simulink model "BD_PAR_AUTO_base_model"  (Simulink 10.3)
settings: Solver=ode1  StartTime=0.0  StopTime=max(cyc_mph(:,1))  FixedStep=1  MaxStep=1  RelTol=1e-3  AbsTol=1e-3
undefined symbols (not defined in the file): acc_dcdc_eff, acc_elec_eff, acc_elec_pwr, acc_mech_eff, acc_mech_pwr, acc_mech_trq, air_cp, amb_tmp, cs_charge_deplete_bool, cs_charge_trq, cs_electric_decel_spd, cs_electric_launch_spd_hi, cs_electric_launch_spd_lo, cs_hi_soc, cs_lo_soc, cs_min_trq_frac, cs_off_trq_frac, cyc_avg_time, cyc_cargo_mass, cyc_elevation_init, cyc_filter_bool, cyc_grade, cyc_mph, enable_sim_stop_distance, enable_sim_stop_max_spd, enable_sim_stop_speed, enable_sim_stop_time, enable_stop, enable_stop_fc, ess_cap_scale, ess_coulombic_eff, ess_init_soc, ess_max_ah_cap, ess_max_volts, ess_min_volts, ess_mod_airflow, ess_mod_cp, ess_mod_init_tmp, ess_module_mass, ess_module_num, ess_on, ess_r_chg, ess_r_dis, ess_res_scale_coef, ess_res_scale_fun, ess_set_tmp, ess_soc, ess_th_calc, ess_th_res_off, ess_th_res_on, ess_tmp, ess_voc, ex_calc, ex_cat_co_frac, ex_cat_ext_cp, ex_cat_ext_emisv, ex_cat_ext_init_tmp, ex_cat_ext_mass, ex_cat_ext_sarea, ex_cat_hc_frac ... (+168)
(part 8 of 15)

== system BD_PAR_AUTO_base_model/<vc> par auto/gearbox control for use w/ AT/shifting1/time since last shift/just shifted ==
  in_1 : Inport
  Memory : Memory  InitialCondition=1
  Relational Operator : RelationalOperator  Operator=~=  RndMeth=Nearest  InputSameDT=on
  out_1 : Outport  InitialOutput=0
  wires:
  in_1/1 -> Memory/1, Relational Operator/2
  Memory/1 -> Relational Operator/1
  Relational Operator/1 -> out_1/1

== system BD_PAR_AUTO_base_model/<vc> par auto/gearbox control for use w/ AT/shifting1/time since last shift/timer ==
  trigger : Inport
  Constant : Constant
  Constant1 : Constant  Value=0
  Constant2 : Constant  Value=0
  Switch : Switch  Threshold=eps
  no-lag Reset Integrator : Subsystem  mask(No-lag Reset Integrator){initval=15}
      mask prompts: initval "Initial Value"
      mask help: No-lag Reset Integrator
      mask Help: Integrates first input using Euler technique.\nAt the time step that input 2 <> zero,\noutput is reset to input 3.
      mask Display: disp('1/s\nw/ reset\nno lag')
  time : Outport  InitialOutput=0
  wires:
  no-lag Reset Integrator/1(out_1) -> Switch/3
  Constant1/1 -> no-lag Reset Integrator/3(in_3)
  Constant/1 -> no-lag Reset Integrator/1(in_1)
  Constant2/1 -> Switch/1
  trigger/1 -> no-lag Reset Integrator/2(in_2), Switch/2
  Switch/1 -> time/1

== system BD_PAR_AUTO_base_model/electric acc loads <acc>/Electrical Accessory Loads v2 <acc>/backward model/electrical accessories (W)/Electrical Accessories: Time Variable ==
  note: (W)
  Constant : Constant  Value=acc_elec_pwr
  Constant1 : Constant  Value=load_on
  Elec Aux Loads 14V Pwr : Subsystem
  Elec Aux Loads HiV Pwr : Subsystem
  Product : Product  InputSameDT=on  RndMeth=Zero  SaturateOnIntegerOverflow=on  OutDataTypeStr=Inherit: Same as first input
  Sum : Sum  Inputs=+++  InputSameDT=on  SaturateOnIntegerOverflow=on  OutDataTypeStr=Inherit: Same as first input
  dcdc converter : Gain  Gain=1/acc_dcdc_eff  SaturateOnIntegerOverflow=on  OutDataTypeStr=Inherit: Same as input  ParamDataTypeStr=Inherit: Same as input
  divide by eff : Gain  Gain=1/acc_elec_eff  SaturateOnIntegerOverflow=on  OutDataTypeStr=Inherit: Same as input  ParamDataTypeStr=Inherit: Same as input
  P_elec_acc : Outport  InitialOutput=0
  wires:
  Elec Aux Loads HiV Pwr/1(Out1) -> Sum/3
  dcdc converter/1 -> Sum/2
  Constant/1 -> Sum/1
  Constant1/1 -> Product/2
  Product/1 -> P_elec_acc/1
  divide by eff/1 -> Product/1
  Sum/1 -> divide by eff/1
  Elec Aux Loads 14V Pwr/1(Out1) -> dcdc converter/1

== system BD_PAR_AUTO_base_model/energy storage <ess>/ess config/energy storage <ess>/ess tmp/Block NOTES ==
  note: This block models the thermal behavior of a battery module with active air cooling.
      | The module is modeled as a single lumped thermal mass.
      | The fan is on whenever the battery temp is > the set temp.

== system BD_PAR_AUTO_base_model/energy storage <ess>/ess config/energy storage <ess>/ess tmp/Tair,ave ==
  Qess_case : Inport
  Qess_case1 : Inport  Port=2
  Enable : EnablePort  StatesWhenEnabling=reset
  Block NOTES : Subsystem
      mask Display: disp('Block\nNOTES')
  Tamb-(Q/mcp)/1 : Fcn  Expr=amb_tmp - (u(1)/(ess_mod_airflow*air_cp))/2
  Tamb-(Q/mcp)/2 : Fcn  Expr=amb_tmp - (u(1)/(ess_mod_airflow*air_cp))/2
  do ex calcs?1 : Constant  Value=ess_th_res_on
  Tair_ave : Outport  OutputWhenDisabled=reset  InitialOutput=amb_tmp
  Th Res : Outport  Port=2  OutputWhenDisabled=reset  InitialOutput=ess_th_res_off
  Tair : Outport  Port=3  InitialOutput=amb_tmp
  wires:
  Tamb-(Q/mcp)/1/1 -> Tair/1
  Qess_case1/1 -> Tamb-(Q/mcp)/1/1
  Tamb-(Q/mcp)/2/1 -> Tair_ave/1
  Qess_case/1 -> Tamb-(Q/mcp)/2/1
  do ex calcs?1/1 -> Th Res/1

== system BD_PAR_AUTO_base_model/energy storage <ess>/ess config/energy storage <ess>/limit power/Limits ==
  SOC  high limited : Inport
  not SOC  low limited : Inport  Port=2
  power req : Inport  Port=3
  power bat limited : Inport  Port=4
  V used : Inport  Port=5
  V mc_min_volts : Inport  Port=6
  V battery (.5Voc) : Inport  Port=7
  V ess_min_volts : Inport  Port=8
  Logical Operator1 : Logic  Operator=NOT  Inputs=1
  Relational Operator{1,3..5} (4 alike) : RelationalOperator  Operator===  RndMeth=Nearest  InputSameDT=on
  limited by battery : Logic
  limited by battery min V : Logic
  limited by motor controller : Logic
  tag scope: ess_minV_limited=global, ess_pwr_limited=global, ess_soc_hi_limited=global, ess_soc_low_limited=global, mc_voltage_limited=global
  wires:
  power bat limited/1 -> Relational Operator1/2
  V mc_min_volts/1 -> Relational Operator3/2
  V used/1 -> Relational Operator3/1, Relational Operator4/1, Relational Operator5/1
  V battery (.5Voc)/1 -> Relational Operator4/2
  V ess_min_volts/1 -> Relational Operator5/2
  limited by motor controller/1 -> [mc_voltage_limited]
  limited by battery/1 -> [ess_pwr_limited]
  limited by battery min V/1 -> [ess_minV_limited]
  Relational Operator3/1 -> limited by motor controller/2
  Relational Operator1/1 -> limited by motor controller/1, limited by battery/1, limited by battery min V/1
  Relational Operator4/1 -> limited by battery/2
  Relational Operator5/1 -> limited by battery min V/2
  power req/1 -> Relational Operator1/1
  Logical Operator1/1 -> [ess_soc_low_limited]
  not SOC  low limited/1 -> Logical Operator1/1
  SOC  high limited/1 -> [ess_soc_hi_limited]

== system BD_PAR_AUTO_base_model/energy storage <ess>/ess config/energy storage <ess>/max pack pwr (W)1/Rchg (ohms)1 ==
  x0 : Inport
  y0 : Inport  Port=2
  Mux : Mux  Inputs=2
  S-function : S-Function  FunctionName=sftable2  Parameters=xindex, yindex, table  SFunctionDeploymentMode=off  EnableBusSupport=off
  table out : Outport  InitialOutput=0
  wires:
  Mux/1 -> S-function/1
  x0/1 -> Mux/1
  S-function/1 -> table out/1
  y0/1 -> Mux/2

== system BD_PAR_AUTO_base_model/energy storage <ess>/ess config/energy storage <ess>/max pack pwr (W)1/Rdis (ohms) ==
  x0 : Inport
  y0 : Inport  Port=2
  Mux : Mux  Inputs=2
  S-function : S-Function  FunctionName=sftable2  Parameters=xindex, yindex, table  SFunctionDeploymentMode=off  EnableBusSupport=off
  table out : Outport  InitialOutput=0
  wires:
  Mux/1 -> S-function/1
  x0/1 -> Mux/1
  S-function/1 -> table out/1
  y0/1 -> Mux/2

== system BD_PAR_AUTO_base_model/energy storage <ess>/ess config/energy storage <ess>/max pack pwr (W)1/VOC (V) ==
  x0 : Inport
  y0 : Inport  Port=2
  Mux : Mux  Inputs=2
  S-function : S-Function  FunctionName=sftable2  Parameters=xindex, yindex, table  SFunctionDeploymentMode=off  EnableBusSupport=off
  table out : Outport  InitialOutput=0
  wires:
  Mux/1 -> S-function/1
  x0/1 -> Mux/1
  S-function/1 -> table out/1
  y0/1 -> Mux/2

== system BD_PAR_AUTO_base_model/energy storage <ess>/ess config/energy storage <ess>/pack Voc, Rint/Rchg (ohms) ==
  x0 : Inport
  y0 : Inport  Port=2
  Mux : Mux  Inputs=2
  S-function : S-Function  FunctionName=sftable2  Parameters=xindex, yindex, table  SFunctionDeploymentMode=off  EnableBusSupport=off
  table out : Outport  InitialOutput=0
  wires:
  y0/1 -> Mux/2
  S-function/1 -> table out/1
  x0/1 -> Mux/1
  Mux/1 -> S-function/1

== system BD_PAR_AUTO_base_model/energy storage <ess>/ess config/energy storage <ess>/pack Voc, Rint/Rdis (ohms) ==
  x0 : Inport
  y0 : Inport  Port=2
  Mux : Mux  Inputs=2
  S-function : S-Function  FunctionName=sftable2  Parameters=xindex, yindex, table  SFunctionDeploymentMode=off  EnableBusSupport=off
  table out : Outport  InitialOutput=0
  wires:
  y0/1 -> Mux/2
  S-function/1 -> table out/1
  x0/1 -> Mux/1
  Mux/1 -> S-function/1

== system BD_PAR_AUTO_base_model/energy storage <ess>/ess config/energy storage <ess>/pack Voc, Rint/VOC (V) ==
  x0 : Inport
  y0 : Inport  Port=2
  Mux : Mux  Inputs=2
  S-function : S-Function  FunctionName=sftable2  Parameters=xindex, yindex, table  SFunctionDeploymentMode=off  EnableBusSupport=off
  table out : Outport  InitialOutput=0
  wires:
  y0/1 -> Mux/2
  S-function/1 -> table out/1
  x0/1 -> Mux/1
  Mux/1 -> S-function/1

== system BD_PAR_AUTO_base_model/fuel converter  <fc>/engine torque/effect of inertia (Nm)/engine inertia as a function of total vehicle inertia (generous approximation)/veh mass calc ==
  Constant : Constant  Value=veh_mass
  Sum : Sum  Inputs=|++  InputSameDT=on  SaturateOnIntegerOverflow=on  OutDataTypeStr=Inherit: Same as first input
  Out1 : Outport
  wires:
  Sum/1 -> Out1/1
  Constant/1 -> Sum/2
  [veh_cargo_mass] -> Sum/1

== system BD_PAR_AUTO_base_model/fuel converter  <fc>/fuel use and EO emis Configurable Subsystem/fuel use and EO emis/HOT engine maps /Block NOTES ==
  note: This block determines the fully hot fuel use, engine-out emissions output rates, exhaust gas mass flow rate,
      | and engine-out exhaust gas temperature as a function of engine output torque and speed.
      | The engine maps (except for exhaust gas temperature) can be scaled using variables fc_spd_scale and
      |  fc_trq_scale; it is recommended that scaling values outside the range of 0.85 to 1.15 be used CAREFULLY.

== system BD_PAR_AUTO_base_model/fuel converter  <fc>/fuel use and EO emis Configurable Subsystem/fuel use and EO emis/HOT engine maps /CO (g/s) ==
  x0 : Inport
  y0 : Inport  Port=2
  Mux : Mux  Inputs=2
  S-function : S-Function  FunctionName=sftable2  Parameters=xindex, yindex, table  SFunctionDeploymentMode=off  EnableBusSupport=off
  table out : Outport  InitialOutput=0
  wires:
  Mux/1 -> S-function/1
  x0/1 -> Mux/1
  S-function/1 -> table out/1
  y0/1 -> Mux/2

== system BD_PAR_AUTO_base_model/fuel converter  <fc>/fuel use and EO emis Configurable Subsystem/fuel use and EO emis/HOT engine maps /HC (g/s) ==
  x0 : Inport
  y0 : Inport  Port=2
  Mux : Mux  Inputs=2
  S-function : S-Function  FunctionName=sftable2  Parameters=xindex, yindex, table  SFunctionDeploymentMode=off  EnableBusSupport=off
  table out : Outport  InitialOutput=0
  wires:
  Mux/1 -> S-function/1
  x0/1 -> Mux/1
  S-function/1 -> table out/1
  y0/1 -> Mux/2

== system BD_PAR_AUTO_base_model/fuel converter  <fc>/fuel use and EO emis Configurable Subsystem/fuel use and EO emis/HOT engine maps /MF,ex (g/s) ==
  x0 : Inport
  y0 : Inport  Port=2
  Mux : Mux  Inputs=2
  S-function : S-Function  FunctionName=sftable2  Parameters=xindex, yindex, table  SFunctionDeploymentMode=off  EnableBusSupport=off
  table out : Outport  InitialOutput=0
  wires:
  Mux/1 -> S-function/1
  x0/1 -> Mux/1
  S-function/1 -> table out/1
  y0/1 -> Mux/2

== system BD_PAR_AUTO_base_model/fuel converter  <fc>/fuel use and EO emis Configurable Subsystem/fuel use and EO emis/HOT engine maps /NOx (g/s) ==
  x0 : Inport
  y0 : Inport  Port=2
  Mux : Mux  Inputs=2
  S-function : S-Function  FunctionName=sftable2  Parameters=xindex, yindex, table  SFunctionDeploymentMode=off  EnableBusSupport=off
  table out : Outport  InitialOutput=0
  wires:
  Mux/1 -> S-function/1
  x0/1 -> Mux/1
  S-function/1 -> table out/1
  y0/1 -> Mux/2

== system BD_PAR_AUTO_base_model/fuel converter  <fc>/fuel use and EO emis Configurable Subsystem/fuel use and EO emis/HOT engine maps /O2 (g/s) ==
  x0 : Inport
  y0 : Inport  Port=2
  Mux : Mux  Inputs=2
  S-function : S-Function  FunctionName=sftable2  Parameters=xindex, yindex, table  SFunctionDeploymentMode=off  EnableBusSupport=off
  table out : Outport  InitialOutput=0
  wires:
  y0/1 -> Mux/2
  S-function/1 -> table out/1
  x0/1 -> Mux/1
  Mux/1 -> S-function/1

== system BD_PAR_AUTO_base_model/fuel converter  <fc>/fuel use and EO emis Configurable Subsystem/fuel use and EO emis/HOT engine maps /PM (g/s) ==
  x0 : Inport
  y0 : Inport  Port=2
  Mux : Mux  Inputs=2
  S-function : S-Function  FunctionName=sftable2  Parameters=xindex, yindex, table  SFunctionDeploymentMode=off  EnableBusSupport=off
  table out : Outport  InitialOutput=0
  wires:
  Mux/1 -> S-function/1
  x0/1 -> Mux/1
  S-function/1 -> table out/1
  y0/1 -> Mux/2

== system BD_PAR_AUTO_base_model/fuel converter  <fc>/fuel use and EO emis Configurable Subsystem/fuel use and EO emis/HOT engine maps /Tex,eo (C) ==
  x0 : Inport
  y0 : Inport  Port=2
  Mux : Mux  Inputs=2
  S-function : S-Function  FunctionName=sftable2  Parameters=xindex, yindex, table  SFunctionDeploymentMode=off  EnableBusSupport=off
  table out : Outport  InitialOutput=0
  wires:
  Mux/1 -> S-function/1
  x0/1 -> Mux/1
  S-function/1 -> table out/1
  y0/1 -> Mux/2

== system BD_PAR_AUTO_base_model/fuel converter  <fc>/fuel use and EO emis Configurable Subsystem/fuel use and EO emis/HOT engine maps /fuel (g/s) ==
  x0 : Inport
  y0 : Inport  Port=2
  Mux : Mux  Inputs=2
  S-function : S-Function  FunctionName=sftable2  Parameters=xindex, yindex, table  SFunctionDeploymentMode=off  EnableBusSupport=off
  table out : Outport  InitialOutput=0
  wires:
  Mux/1 -> S-function/1
  x0/1 -> Mux/1
  S-function/1 -> table out/1
  y0/1 -> Mux/2

== system BD_PAR_AUTO_base_model/fuel converter  <fc>/fuel use and EO emis Configurable Subsystem/fuel use and EO emis/fc temp/Block NOTES ==
  note: This block models the thermal behavior internal combustion engine (ICE).
      | Emphasis is on the coolant since this temperature is used to correct engine
      | fuel use.

== system BD_PAR_AUTO_base_model/fuel converter  <fc>/fuel use and EO emis Configurable Subsystem/fuel use and EO emis/fc temp/fc coolant ==
  Tcl : Inport
  "Qfc_i " : Inport  Port=2
  Enable : EnablePort  StatesWhenEnabling=reset
  Constant : Constant  Value=fc_tstat
  Product1 : Product  InputSameDT=on  RndMeth=Zero  SaturateOnIntegerOverflow=on  OutDataTypeStr=Inherit: Same as first input
  Qhtr : Fcn  Expr=fc_cl2h_eff*fc_h_air_flow*air_cp*(u - amb_tmp)
  Qi : Sum  Inputs=-+  InputSameDT=on  SaturateOnIntegerOverflow=on  OutDataTypeStr=Inherit: Same as first input
  Relational Operator : RelationalOperator  Operator=<=  RndMeth=Nearest  InputSameDT=on
  Qfc_rad : Outport  OutputWhenDisabled=reset  InitialOutput=0
  Qfc_htr : Outport  Port=2  OutputWhenDisabled=reset  InitialOutput=0
  wires:
  Tcl/1 -> Qhtr/1, Relational Operator/2
  Relational Operator/1 -> Product1/1
  Constant/1 -> Relational Operator/1
  Product1/1 -> Qfc_rad/1
  "Qfc_i "/1 -> Qi/2
  Qhtr/1 -> Qi/1, Qfc_htr/1
  Qi/1 -> Product1/2

== system BD_PAR_AUTO_base_model/fuel converter  <fc>/fuel use and EO emis Configurable Subsystem/fuel use and EO emis/fc temp/fc mass heat flow ==
  veh spd : Inport
  fc_temp : Inport  Port=2
  Block NOTES : Subsystem
      mask Display: disp('Block\nNOTES')
  Mux{3..6,9..10} (6 alike) : Mux  Inputs=2
  Qh : Sum  Inputs=-++  InputSameDT=on  SaturateOnIntegerOverflow=on  OutDataTypeStr=Inherit: Same as first input
  Qh2a,r : Fcn  Expr=fc_hood_emisv*(5.67e-8)*fc_hood_sarea*((amb_tmp+273)^4 - (u(4)+273)^4)
  Qh2a,v : Fcn  Expr=u(2)*fc_hood_sarea*u(1)
  Qh2x : Sum  Inputs=+++  InputSameDT=on  SaturateOnIntegerOverflow=on  OutDataTypeStr=Inherit: Same as first input
  Qh2x,r : Fcn  Expr=fc_emisv*(5.67e-8)*fc_ext_sarea*fc_pwr_scale^0.67*((u(4)+273)^4 - (u(3)+273)^4)
  Qh2x,r1 : Fcn  Expr=fc_emisv*(5.67e-8)*(0.5*fc_ext_sarea*fc_pwr_scale^0.67)*((amb_tmp+273)^4 - (u(3)+273)^4)
  Qh2x,v : Fcn  Expr=u(2)*fc_ext_sarea*fc_pwr_scale^0.67*u(1)
  Qh2x,v1 : Fcn  Expr=u(2)*(0.5*fc_ext_sarea*fc_pwr_scale^0.67)*u(1)
  Qi : Sum  Inputs=-+  InputSameDT=on  SaturateOnIntegerOverflow=on  OutDataTypeStr=Inherit: Same as first input
  Qi2c,c : Fcn  Expr=fc_c2i_th_cond*(u(2) - u(1))
  Qp2a,v5 : Fcn  Expr=u(4)-u(3)
  Qp2a,v6 : Fcn  Expr=amb_tmp-u(4)
  Qp2a,v7 : Fcn  Expr=amb_tmp-u(3)
  Qx : Sum  Inputs=-++  InputSameDT=on  SaturateOnIntegerOverflow=on  OutDataTypeStr=Inherit: Same as first input
  Qx1 : Sum  InputSameDT=on  SaturateOnIntegerOverflow=on  OutDataTypeStr=Inherit: Same as first input
  Qx2i,c : Fcn  Expr=fc_i2x_th_cond*(u(3) - u(2))
  Qx2p,c : Fcn  Expr=fc_h2x_th_cond*(u(4) - u(3))
  Va/Vv : Gain  Gain=0.5  SaturateOnIntegerOverflow=on  OutDataTypeStr=Inherit: Same as input  ParamDataTypeStr=Inherit: Same as input
  Va/Vv1 : Gain  Gain=0.5  SaturateOnIntegerOverflow=on  OutDataTypeStr=Inherit: Same as input  ParamDataTypeStr=Inherit: Same as input
  h_h2a : Fcn  Expr=10 + 6*(abs(u(1))/1000)^0.3 + 60*(abs(u(2))/30)^0.6
  h_h2x : Fcn  Expr=6 + 6*((abs(u(1))/1000))^0.3 + 60*(abs(u(2))/30)^0.6
  h_h2x1 : Fcn  Expr=6 + 6*((abs(u(1))/1000))^0.3 + 60*(abs(u(2))/30)^0.6
  Qfc_c : Outport
  Qfc_i : Outport  Port=2
  Qfc_x : Outport  Port=3
  Qfc_h : Outport  Port=4
  wires:
  Mux10/1 -> Qh2x,v1/1
  Mux9/1 -> h_h2x1/1
  Qp2a,v7/1 -> Mux9/1, Mux10/1
  h_h2x1/1 -> Mux10/2
  Va/Vv1/1 -> Mux9/2
  Mux4/1 -> Qh2x,v/1
  Mux3/1 -> h_h2x/1
  Qp2a,v5/1 -> Mux3/1, Mux4/1
  h_h2x/1 -> Mux4/2
  veh spd/1 -> Va/Vv/1, Mux5/2, Va/Vv1/1
  Va/Vv/1 -> Mux3/2
  Qi2c,c/1 -> Qfc_c/1, Qi/1
  fc_temp/1 -> Qx2p,c/1, Qh2x,r/1, Qp2a,v7/1, Qp2a,v6/1, Qh2a,r/1, Qh2x,r1/1, Qp2a,v5/1, Qx2i,c/1, Qi2c,c/1
  Qx2i,c/1 -> Qi/2, Qx/1
  Qi/1 -> Qfc_i/1
  Qx/1 -> Qfc_x/1
  Qh2x/1 -> Qx/2, Qh/1
  Qh/1 -> Qfc_h/1
  Mux6/1 -> Qh2a,v/1
  Mux5/1 -> h_h2a/1
  Qp2a,v6/1 -> Mux5/1, Mux6/1
  h_h2a/1 -> Mux6/2
  Qx1/1 -> Qx/3
  Qh2x,v/1 -> Qh2x/2
  Qx2p,c/1 -> Qh2x/1
  Qh2x,r1/1 -> Qx1/2
  Qh2x,v1/1 -> Qx1/1
  Qh2a,r/1 -> Qh/3
  Qh2a,v/1 -> Qh/2
  Qh2x,r/1 -> Qh2x/3

== system BD_PAR_AUTO_base_model/fuel converter  <fc>/fuel use and EO emis Configurable Subsystem/fuel use and EO emis/fc temp/old fc coolant  temp. (C) ==
  fc on? : Inport
  veh spd : Inport  Port=2
  Block NOTES : Subsystem
      mask Display: disp('Block\nNOTES')
  Mux : Mux
  TEC : Integrator  InitialCondition=fc_i_init_tmp
  compute engine dT/dt : Fcn  Expr=1.1*u[1]*(-u[2]/218)*(95-u[4])+(1-u[1])*u[3]*(u[4]-amb_tmp)
  gamma (takes v as input) : Fcn  Expr=(-8.22e-5*u+8.09e-6*4-1.45e-4)*.45
  log(1-40/75) : Constant  Value=-0.7621
  fc coolant  temp (C) : Outport  InitialOutput=0
  wires:
  compute engine dT/dt/1 -> TEC/1
  gamma (takes v as input)/1 -> Mux/3
  log(1-40/75)/1 -> Mux/2
  Mux/1 -> compute engine dT/dt/1
  fc on?/1 -> Mux/1
  veh spd/1 -> gamma (takes v as input)/1
  TEC/1 -> fc coolant  temp (C)/1, Mux/4

== system BD_PAR_AUTO_base_model/fuel converter  <fc>/fuel use and EO emis Configurable Subsystem/fuel use and EO emis/fc temp correct/fc temp correct Constant Correction Factors (Equation Based) ==
  Coolant T (C) : Inport
  HOT fuel use (g/s) : Inport  Port=2
  HOT emis (g/s) : Inport  Port=3
  Enable : EnablePort  StatesWhenEnabling=reset
  Block NOTES : Subsystem
      mask Display: disp('Block\nNOTES')
  CO cold/hot : Fcn  Expr=2.13*pow(u,4.26)+1
  HC cold/hot : Fcn  Expr=8.05*pow(u,9.46)+1
  Mux : Mux
  NOx cold/hot : Fcn  Expr=0.51*pow(u,1.37)+1
  PM cold/hot : Fcn  Expr=5.14*pow(u,17.04)+1
  Product : Product  InputSameDT=on  RndMeth=Zero  SaturateOnIntegerOverflow=on  OutDataTypeStr=Inherit: Same as first input
  Product1 : Product  InputSameDT=on  RndMeth=Zero  SaturateOnIntegerOverflow=on  OutDataTypeStr=Inherit: Same as first input
  Saturation : Saturate  UpperLimit=1  LowerLimit=0
  fuel cold/hot : Fcn  Expr=0.1*pow(u,0.65)+1
  lambda : Fcn  Expr=(fc_tstat-u)/(fc_tstat-20)
  fuel use (g/s) : Outport  OutputWhenDisabled=reset  InitialOutput=0
  EO emis (g/s) : Outport  Port=2  OutputWhenDisabled=reset  InitialOutput=0
  wires:
  PM cold/hot/1 -> Mux/4
  NOx cold/hot/1 -> Mux/3
  HC cold/hot/1 -> Mux/1
  Saturation/1 -> CO cold/hot/1, HC cold/hot/1, fuel cold/hot/1, NOx cold/hot/1, PM cold/hot/1
  lambda/1 -> Saturation/1
  Mux/1 -> Product/1
  fuel cold/hot/1 -> Product1/2
  Product/1 -> EO emis (g/s)/1
  CO cold/hot/1 -> Mux/2
  Product1/1 -> fuel use (g/s)/1
  HOT fuel use (g/s)/1 -> Product1/1
  Coolant T (C)/1 -> lambda/1
  HOT emis (g/s)/1 -> Product/2

== system BD_PAR_AUTO_base_model/fuel converter  <fc>/fuel use and EO emis Configurable Subsystem/fuel use and EO emis/fc temp correct/fc temp correct Variable Correction Factors (Map Based) ==
  Coolant T (C) : Inport
  HOT fuel use (g/s) : Inport  Port=2
  HOT emis (g/s) : Inport  Port=3
  T (Nm) : Inport  Port=4
  w (rad/s) : Inport  Port=5
  Enable : EnablePort  StatesWhenEnabling=reset
  (Thot-Temp) -------------------- (Thot-Tcold) : Fcn  Expr=(fc_tstat-u)/(fc_tstat-fc_cold_tmp)
  CO factor cold-to-hot : Subsystem  mask(2-D Table Lookup){xindex=fc_map_spd*fc_spd_scale, yindex=fc_map_trq*fc_trq_scale, table=fc_co_map_c2h}
      mask prompts: xindex "X Index"; yindex "Y Index"
      mask help:
      | Two Dimensional Table Lookup
      | The first input corresponds to X Index and the second input corresponds to the Y Index
      mask init:
      | sftab2chk(xindex,yindex,table);
      mask Help: This block returns a linearly interpolated intersection from the table using the X index (which corresponds to the rows of the table) and the Y index (which corresponds to the columns of the table).  Extrapolation is used.
      mask Display: plot(-10,-10,110,110,[90,50,10],[90,40,30],[90,50,10],[50,26,20],[90,50,10],[22,13,10])
  HC factor cold-to-hot : Subsystem  mask(2-D Table Lookup){xindex=fc_map_spd*fc_spd_scale, yindex=fc_map_trq*fc_trq_scale, table=fc_hc_map_c2h}
      mask prompts: xindex "X Index"; yindex "Y Index"
      mask help:
      | Two Dimensional Table Lookup
      | The first input corresponds to X Index and the second input corresponds to the Y Index
      mask init:
      | sftab2chk(xindex,yindex,table);
      mask Help: This block returns a linearly interpolated intersection from the table using the X index (which corresponds to the rows of the table) and the Y index (which corresponds to the columns of the table).  Extrapolation is used.
      mask Display: plot(-10,-10,110,110,[90,50,10],[90,40,30],[90,50,10],[50,26,20],[90,50,10],[22,13,10])
  Mux{1..5} (5 alike) : Mux  Inputs=2
  Mux6 : Mux
  NOx factor cold-to-hot : Subsystem  mask(2-D Table Lookup){xindex=fc_map_spd*fc_spd_scale, yindex=fc_map_trq*fc_trq_scale, table=fc_nox_map_c2h}
      mask prompts: xindex "X Index"; yindex "Y Index"
      mask help:
      | Two Dimensional Table Lookup
      | The first input corresponds to X Index and the second input corresponds to the Y Index
      mask init:
      | sftab2chk(xindex,yindex,table);
      mask Help: This block returns a linearly interpolated intersection from the table using the X index (which corresponds to the rows of the table) and the Y index (which corresponds to the columns of the table).  Extrapolation is used.
      mask Display: plot(-10,-10,110,110,[90,50,10],[90,40,30],[90,50,10],[50,26,20],[90,50,10],[22,13,10])
  PM factor cold-to-hot : Subsystem  mask(2-D Table Lookup){xindex=fc_map_spd*fc_spd_scale, yindex=fc_map_trq*fc_trq_scale, table=fc_pm_map_c2h}
      mask prompts: xindex "X Index"; yindex "Y Index"
      mask help:
      | Two Dimensional Table Lookup
      | The first input corresponds to X Index and the second input corresponds to the Y Index
      mask init:
      | sftab2chk(xindex,yindex,table);
      mask Help: This block returns a linearly interpolated intersection from the table using the X index (which corresponds to the rows of the table) and the Y index (which corresponds to the columns of the table).  Extrapolation is used.
      mask Display: plot(-10,-10,110,110,[90,50,10],[90,40,30],[90,50,10],[50,26,20],[90,50,10],[22,13,10])
  Product : Product  InputSameDT=on  RndMeth=Zero  SaturateOnIntegerOverflow=on  OutDataTypeStr=Inherit: Same as first input
  Product1 : Product  InputSameDT=on  RndMeth=Zero  SaturateOnIntegerOverflow=on  OutDataTypeStr=Inherit: Same as first input
  Saturation1 : Saturate  UpperLimit=max(fc_map_trq*fc_trq_scale)  LowerLimit=min(fc_map_trq*fc_trq_scale)
  Saturation2 : Saturate  UpperLimit=max(fc_map_spd*fc_spd_scale)  LowerLimit=min(fc_map_spd*fc_spd_scale)
  cold/hot =1+(factor-1) *Temp_ratio{,1..4} (5 alike) : Fcn  Expr=1+(u[2]-1)*u[1]
  fuel factor cold-to-hot : Subsystem  mask(2-D Table Lookup){xindex=fc_map_spd*fc_spd_scale, yindex=fc_map_trq*fc_trq_scale, table=fc_fuel_map_c2h}
      mask prompts: xindex "X Index"; yindex "Y Index"
      mask help:
      | Two Dimensional Table Lookup
      | The first input corresponds to X Index and the second input corresponds to the Y Index
      mask init:
      | sftab2chk(xindex,yindex,table);
      mask Help: This block returns a linearly interpolated intersection from the table using the X index (which corresponds to the rows of the table) and the Y index (which corresponds to the columns of the table).  Extrapolation is used.
      mask Display: plot(-10,-10,110,110,[90,50,10],[90,40,30],[90,50,10],[50,26,20],[90,50,10],[22,13,10])
  limit to data limits : Saturate  UpperLimit=1  LowerLimit=0
  fuel use (g/s) : Outport  OutputWhenDisabled=reset  InitialOutput=0
  EO emis (g/s) : Outport  Port=2  OutputWhenDisabled=reset  InitialOutput=0
  wires:
  cold/hot =1+(factor-1) *Temp_ratio4/1 -> Mux6/4
  cold/hot =1+(factor-1) *Temp_ratio3/1 -> Mux6/3
  cold/hot =1+(factor-1) *Temp_ratio2/1 -> Mux6/2
  cold/hot =1+(factor-1) *Temp_ratio1/1 -> Mux6/1
  cold/hot =1+(factor-1) *Temp_ratio/1 -> Product1/2
  limit to data limits/1 -> Mux5/1, Mux4/1, Mux3/1, Mux2/1, Mux1/1
  (Thot-Temp) -------------------- (Thot-Tcold)/1 -> limit to data limits/1
  Mux6/1 -> Product/1
  w (rad/s)/1 -> Saturation2/1
  T (Nm)/1 -> Saturation1/1
  HOT emis (g/s)/1 -> Product/2
  Product/1 -> EO emis (g/s)/1
  Product1/1 -> fuel use (g/s)/1
  Mux5/1 -> cold/hot =1+(factor-1) *Temp_ratio4/1
  Mux4/1 -> cold/hot =1+(factor-1) *Temp_ratio3/1
  Mux3/1 -> cold/hot =1+(factor-1) *Temp_ratio2/1
  Mux2/1 -> cold/hot =1+(factor-1) *Temp_ratio1/1
  PM factor cold-to-hot/1(table out) -> Mux5/2
  NOx factor cold-to-hot/1(table out) -> Mux4/2
  CO factor cold-to-hot/1(table out) -> Mux3/2
  HC factor cold-to-hot/1(table out) -> Mux2/2
  Mux1/1 -> cold/hot =1+(factor-1) *Temp_ratio/1
  fuel factor cold-to-hot/1(table out) -> Mux1/2
  Coolant T (C)/1 -> (Thot-Temp) -------------------- (Thot-Tcold)/1
  Saturation1/1 -> PM factor cold-to-hot/2(y0), NOx factor cold-to-hot/2(y0), CO factor cold-to-hot/2(y0), HC factor cold-to-hot/2(y0), fuel factor cold-to-hot/2(y0)
  Saturation2/1 -> PM factor cold-to-hot/1(x0), NOx factor cold-to-hot/1(x0), CO factor cold-to-hot/1(x0), HC factor cold-to-hot/1(x0), fuel factor cold-to-hot/1(x0)
  HOT fuel use (g/s)/1 -> Product1/1

== system BD_PAR_AUTO_base_model/mechanical accessory loads <acc>/Mechanical Accessory Loads v2 <acc>/backward model/mechanical accessories (Nm)/Mechanical Accessories: Const Mech Var Elect ==
  note: (W)
  note: (Nm)
  note: engine shaft speed
  w_APU : Inport
  Constant : Constant  Value=acc_mech_pwr
  Constant1 : Constant  Value=acc_mech_trq
  Constant2 : Constant  Value=acc_elec_pwr
  Constant3 : Constant  Value=load_on
  Elec Aux Loads 14V Pwr : Subsystem
  Elec Aux Loads HiV Pwr : Subsystem
  Ground : Ground
  Mux : Mux  Inputs=3
  Product : Product  InputSameDT=on  RndMeth=Zero  SaturateOnIntegerOverflow=on  OutDataTypeStr=Inherit: Same as first input
  Sum1 : Sum  Inputs=+++  InputSameDT=on  SaturateOnIntegerOverflow=on  OutDataTypeStr=Inherit: Same as first input
  accessory mechanical torque and power calcs (Nm) : Subsystem  mask{load_on=load_on}
      mask prompts: load_on "FLAG: (1= don't use acc_elec_pwr; 0= use acc_elec_pwr here)"
  dcdc converter : Gain  Gain=1/acc_dcdc_eff  SaturateOnIntegerOverflow=on  OutDataTypeStr=Inherit: Same as input  ParamDataTypeStr=Inherit: Same as input
  T_acc : Outport  InitialOutput=0
  P_mech_acc : Outport  Port=2  InitialOutput=0
  probes : Outport  Port=3  InitialOutput=0
  wires:
  Elec Aux Loads HiV Pwr/1(Out1) -> Sum1/3
  dcdc converter/1 -> Sum1/2
  Sum1/1 -> Product/1
  Constant2/1 -> Sum1/1
  Elec Aux Loads 14V Pwr/1(Out1) -> dcdc converter/1
  Ground/1 -> probes/1
  Constant3/1 -> Product/2
  Product/1 -> Mux/3
  Constant1/1 -> Mux/2
  Constant/1 -> Mux/1
  Mux/1 -> accessory mechanical torque and power calcs (Nm)/2("accessorie loads \"function\" return values")
  accessory mechanical torque and power calcs (Nm)/2(P_acc) -> P_mech_acc/1
  accessory mechanical torque and power calcs (Nm)/1(T_acc) -> T_acc/1
  w_APU/1 -> accessory mechanical torque and power calcs (Nm)/1(w_APU)

== system BD_PAR_AUTO_base_model/vehicle <veh>/record achieved force outputs/rolling resistance force/force req'd to overcome rolling resistance (N)/current veh mass ==
  Constant3 : Constant  Value=veh_mass
  Sum1 : Sum  Inputs=|++  SaturateOnIntegerOverflow=on
  Out1 : Outport
  wires:
  Constant3/1 -> Sum1/1
  [veh_cargo_mass] -> Sum1/2
  Sum1/1 -> Out1/1

== system BD_PAR_AUTO_base_model/vehicle <veh>/vehicle speed/vehicle speed (m/s)/b/current veh mass ==
  Constant3 : Constant  Value=veh_mass
  Sum1 : Sum  Inputs=|++  SaturateOnIntegerOverflow=on
  Out1 : Outport
  wires:
  Constant3/1 -> Sum1/1
  [veh_cargo_mass] -> Sum1/2
  Sum1/1 -> Out1/1

== system BD_PAR_AUTO_base_model/vehicle <veh>/vehicle speed/vehicle speed (m/s)/b/current veh mass1 ==
  Constant3 : Constant  Value=veh_mass
  Sum1 : Sum  Inputs=|++  SaturateOnIntegerOverflow=on
  Out1 : Outport
  wires:
  Constant3/1 -> Sum1/1
  [veh_cargo_mass] -> Sum1/2
  Sum1/1 -> Out1/1

== system BD_PAR_AUTO_base_model/vehicle <veh>/vehicle speed/vehicle speed (m/s)/c/current veh mass ==
  Constant3 : Constant  Value=veh_mass
  Sum1 : Sum  Inputs=|++  SaturateOnIntegerOverflow=on
  Out1 : Outport
  wires:
  Constant3/1 -> Sum1/1
  [veh_cargo_mass] -> Sum1/2
  Sum1/1 -> Out1/1

== system BD_PAR_AUTO_base_model/vehicle <veh>/vehicle speed/vehicle speed (m/s)/c/current veh mass1 ==
  Constant3 : Constant  Value=veh_mass
  Sum1 : Sum  Inputs=|++  SaturateOnIntegerOverflow=on
  Out1 : Outport
  wires:
  Constant3/1 -> Sum1/1
  [veh_cargo_mass] -> Sum1/2
  Sum1/1 -> Out1/1

== system BD_PAR_AUTO_base_model/<vc> par auto/config traction control/traction control 2 axle/apply tire traction limit to req'd speed (m/s)/rear slip terms/current  veh mass (kg) ==
  Constant12 : Constant  Value=veh_mass
  Sum8 : Sum  Inputs=|++  InputSameDT=on  SaturateOnIntegerOverflow=on  OutDataTypeStr=Inherit: Same as first input
  Out1 : Outport
  wires:
  Constant12/1 -> Sum8/2
  [veh_cargo_mass] -> Sum8/1
  Sum8/1 -> Out1/1

== system BD_PAR_AUTO_base_model/<vc> par auto/config traction control/traction control 2 axle/enforce max.  front axle tractive force  due to slip (N)/front/current veh mass (kg) ==
  Constant12 : Constant  Value=veh_mass
  Sum8 : Sum  Inputs=|++  InputSameDT=on  SaturateOnIntegerOverflow=on  OutDataTypeStr=Inherit: Same as first input
  Out1 : Outport
  wires:
  Constant12/1 -> Sum8/2
  [veh_cargo_mass] -> Sum8/1
  Sum8/1 -> Out1/1

== system BD_PAR_AUTO_base_model/<vc> par auto/config traction control/traction control 2 axle/enforce max.  front axle tractive force  due to slip (N)/rear/current veh mass (kg) ==
  Constant12 : Constant  Value=veh_mass
  Sum8 : Sum  Inputs=|++  InputSameDT=on  SaturateOnIntegerOverflow=on  OutDataTypeStr=Inherit: Same as first input
  Out1 : Outport
  wires:
  Constant12/1 -> Sum8/2
  [veh_cargo_mass] -> Sum8/1
  Sum8/1 -> Out1/1

== system BD_PAR_AUTO_base_model/<vc> par auto/gearbox control for use w/ AT/Speed Dependent Shifting/shifting/time since last shift/just shifted ==
  in_1 : Inport
  Memory : Memory  InitialCondition=1
  Relational Operator : RelationalOperator  Operator=~=  RndMeth=Nearest  InputSameDT=on
  out_1 : Outport  InitialOutput=0
  wires:
  in_1/1 -> Memory/1, Relational Operator/2
  Memory/1 -> Relational Operator/1
  Relational Operator/1 -> out_1/1

== system BD_PAR_AUTO_base_model/<vc> par auto/gearbox control for use w/ AT/Speed Dependent Shifting/shifting/time since last shift/timer ==
  trigger : Inport
  Constant : Constant
  Constant1 : Constant  Value=0
  Constant2 : Constant  Value=0
  Switch : Switch  Threshold=eps
  no-lag Reset Integrator : Subsystem  mask(No-lag Reset Integrator){initval=15}
      mask prompts: initval "Initial Value"
      mask help: No-lag Reset Integrator
      mask Help: Integrates first input using Euler technique.\nAt the time step that input 2 <> zero,\noutput is reset to input 3.
      mask Display: disp('1/s\nw/ reset\nno lag')
  time : Outport  InitialOutput=0
  wires:
  no-lag Reset Integrator/1(out_1) -> Switch/3
  Constant1/1 -> no-lag Reset Integrator/3(in_3)
  Constant/1 -> no-lag Reset Integrator/1(in_1)
  Constant2/1 -> Switch/1
  trigger/1 -> no-lag Reset Integrator/2(in_2), Switch/2
  Switch/1 -> time/1

== system BD_PAR_AUTO_base_model/<vc> par auto/gearbox control for use w/ AT/Speed Dependent Shifting/shifting1/time since last shift/just shifted ==
  in_1 : Inport
  Memory : Memory  InitialCondition=1
  Relational Operator : RelationalOperator  Operator=~=  RndMeth=Nearest  InputSameDT=on
  out_1 : Outport  InitialOutput=0
  wires:
  in_1/1 -> Memory/1, Relational Operator/2
  Memory/1 -> Relational Operator/1
  Relational Operator/1 -> out_1/1

== system BD_PAR_AUTO_base_model/<vc> par auto/gearbox control for use w/ AT/Speed Dependent Shifting/shifting1/time since last shift/timer ==
  trigger : Inport
  Constant : Constant
  Constant1 : Constant  Value=0
  Constant2 : Constant  Value=0
  Switch : Switch  Threshold=eps
  no-lag Reset Integrator : Subsystem  mask(No-lag Reset Integrator){initval=15}
      mask prompts: initval "Initial Value"
      mask help: No-lag Reset Integrator
      mask Help: Integrates first input using Euler technique.\nAt the time step that input 2 <> zero,\noutput is reset to input 3.
      mask Display: disp('1/s\nw/ reset\nno lag')
  time : Outport  InitialOutput=0
  wires:
  no-lag Reset Integrator/1(out_1) -> Switch/3
  Constant1/1 -> no-lag Reset Integrator/3(in_3)
  Constant/1 -> no-lag Reset Integrator/1(in_1)
  Constant2/1 -> Switch/1
  trigger/1 -> no-lag Reset Integrator/2(in_2), Switch/2
  Switch/1 -> time/1

== system BD_PAR_AUTO_base_model/<vc> par auto/gearbox control for use w/ AT/shifting1/time since last shift/timer/no-lag Reset Integrator ==
  in_1 : Inport
  in_2 : Inport  Port=2
  in_3 : Inport  Port=3
  Constant : Constant  Value=0
  Memory : Memory  InitialCondition=initval
  Product : Product  InputSameDT=on  RndMeth=Zero  SaturateOnIntegerOverflow=on  OutDataTypeStr=Inherit: Same as first input
  Sum : Sum  InputSameDT=on  SaturateOnIntegerOverflow=on  OutDataTypeStr=Inherit: Same as first input
  Switch : Switch  Threshold=eps
  dt : Subsystem
  in_2==0 : RelationalOperator  Operator===  RndMeth=Nearest  InputSameDT=on
  out_1 : Outport  InitialOutput=0
  wires:
  Constant/1 -> in_2==0/2
  in_2==0/1 -> Switch/2
  Switch/1 -> Memory/1, out_1/1
  Sum/1 -> Switch/1
  Memory/1 -> Sum/1
  Product/1 -> Sum/2
  dt/1(out_1) -> Product/1
  in_1/1 -> Product/2
  in_2/1 -> in_2==0/1
  in_3/1 -> Switch/3

== system BD_PAR_AUTO_base_model/electric acc loads <acc>/Electrical Accessory Loads v2 <acc>/backward model/electrical accessories (W)/Electrical Accessories: Time Variable/Elec Aux Loads 14V Pwr ==
  BrakeLights : Subsystem
  Constant : Constant  Value=0
  Constant1 : Constant  Value=vinf.AuxLoadsOn
  Engine : Subsystem
  ExternalLights : Subsystem
  FrontHVAC : Subsystem
  FrontWipers : Subsystem
  HeatedSeats : Subsystem
  Misc : Subsystem
  RadiatorCoolingFan : Subsystem
  Radio : Subsystem
  RearDefrost : Subsystem
  RearHVAC : Subsystem
  RearWipers : Subsystem
  Starter : Subsystem
  Sum : Sum  Inputs=++++++++++++++  InputSameDT=on  SaturateOnIntegerOverflow=on  OutDataTypeStr=Inherit: Same as first input
  Switch : Switch  Threshold=.5
  TurnSignals : Subsystem
  Out1 : Outport
  wires:
  Switch/1 -> Out1/1
  Sum/1 -> Switch/1
  Constant/1 -> Switch/3
  Constant1/1 -> Switch/2
  RearDefrost/1(Out1) -> Sum/1
  HeatedSeats/1(Out1) -> Sum/2
  Radio/1(Out1) -> Sum/3
  RearWipers/1(Out1) -> Sum/4
  FrontWipers/1(Out1) -> Sum/5
  TurnSignals/1(Out1) -> Sum/6
  Misc/1(Out1) -> Sum/7
  FrontHVAC/1(Out1) -> Sum/8
  RearHVAC/1(Out1) -> Sum/9
  Engine/1(Out1) -> Sum/10
  ExternalLights/1(Out1) -> Sum/11
  RadiatorCoolingFan/1(Out1) -> Sum/12
  BrakeLights/1(Out1) -> Sum/13
  Starter/1(Out1) -> Sum/14

== system BD_PAR_AUTO_base_model/electric acc loads <acc>/Electrical Accessory Loads v2 <acc>/backward model/electrical accessories (W)/Electrical Accessories: Time Variable/Elec Aux Loads HiV Pwr ==
  Constant : Constant  Value=0
  Constant1 : Constant  Value=vinf.AuxLoadsOn
  CurrentLoad1 : Subsystem
  PowerLoad1 : Subsystem
  PowerLoad2 : Subsystem
  PowerLoad3 : Subsystem
  SpeedLoad1 : Subsystem
  Starter : Subsystem
  Sum : Sum  Inputs=++++++  InputSameDT=on  SaturateOnIntegerOverflow=on  OutDataTypeStr=Inherit: Same as first input
  Switch : Switch  Threshold=.5
  Out1 : Outport
  wires:
  Sum/1 -> Switch/1
  Starter/1(Out1) -> Sum/6
  SpeedLoad1/1(Out1) -> Sum/5
  CurrentLoad1/1(Out1) -> Sum/4
  PowerLoad3/1(Out1) -> Sum/3
  PowerLoad2/1(Out1) -> Sum/2
  PowerLoad1/1(Out1) -> Sum/1
  Constant1/1 -> Switch/2
  Constant/1 -> Switch/3
  Switch/1 -> Out1/1

== system BD_PAR_AUTO_base_model/energy storage <ess>/ess config/energy storage <ess>/ess tmp/Tair,ave/Block NOTES ==
  note: This block determins the average temperature of the cooling air over the module.

== system BD_PAR_AUTO_base_model/fuel converter  <fc>/fuel use and EO emis Configurable Subsystem/fuel use and EO emis/fc temp/fc mass heat flow/Block NOTES ==
  note: FUEL CONVERTER MASS HEAT LOSS
      | This block models the heat loss from a fuel converter (such as an IC engine).
      | Convection (as a function of vehicle speed), radiation, and conduction effects are included.
      | Engine cylinder (c), interior (i), exterior (x) and hood (h)
      | heat flows are estimated based on the temperatures from the previous iteration.

== system BD_PAR_AUTO_base_model/fuel converter  <fc>/fuel use and EO emis Configurable Subsystem/fuel use and EO emis/fc temp/old fc coolant  temp. (C)/Block NOTES ==
  note: This block computes engine coolant temperature,
      | assuming that it asymptotically approaches its maximum
      | temperature when the engine is on, and asymptotically
      | approaches the ambient temperature when the engine
      | is off.  Temperatue rise rate is assumed to be a function
      | only of current engine coolant temperature, and the fall
      | rate is also a function of vehicle speed and ambient temperature.
      | There is no dependence on engine load or speed.

== system BD_PAR_AUTO_base_model/fuel converter  <fc>/fuel use and EO emis Configurable Subsystem/fuel use and EO emis/fc temp correct/fc temp correct Constant Correction Factors (Equation Based)/Block NOTES ==
  note: This block determines actual fuel use and engine-out emissions
      | given the fully hot values and the engine coolant temperature.
      | The correlations used here were developed at NREL using
      | Hot and Cold Engine data collected
      | at Oak Ridge National Laboratory.

== system BD_PAR_AUTO_base_model/fuel converter  <fc>/fuel use and EO emis Configurable Subsystem/fuel use and EO emis/fc temp correct/fc temp correct Variable Correction Factors (Map Based)/CO factor cold-to-hot ==
  x0 : Inport
  y0 : Inport  Port=2
  Mux : Mux  Inputs=2
  S-function : S-Function  FunctionName=sftable2  Parameters=xindex, yindex, table  SFunctionDeploymentMode=off  EnableBusSupport=off
  table out : Outport  InitialOutput=0
  wires:
  y0/1 -> Mux/2
  S-function/1 -> table out/1
  x0/1 -> Mux/1
  Mux/1 -> S-function/1

== system BD_PAR_AUTO_base_model/fuel converter  <fc>/fuel use and EO emis Configurable Subsystem/fuel use and EO emis/fc temp correct/fc temp correct Variable Correction Factors (Map Based)/HC factor cold-to-hot ==
  x0 : Inport
  y0 : Inport  Port=2
  Mux : Mux  Inputs=2
  S-function : S-Function  FunctionName=sftable2  Parameters=xindex, yindex, table  SFunctionDeploymentMode=off  EnableBusSupport=off
  table out : Outport  InitialOutput=0
  wires:
  y0/1 -> Mux/2
  S-function/1 -> table out/1
  x0/1 -> Mux/1
  Mux/1 -> S-function/1

== system BD_PAR_AUTO_base_model/fuel converter  <fc>/fuel use and EO emis Configurable Subsystem/fuel use and EO emis/fc temp correct/fc temp correct Variable Correction Factors (Map Based)/NOx factor cold-to-hot ==
  x0 : Inport
  y0 : Inport  Port=2
  Mux : Mux  Inputs=2
  S-function : S-Function  FunctionName=sftable2  Parameters=xindex, yindex, table  SFunctionDeploymentMode=off  EnableBusSupport=off
  table out : Outport  InitialOutput=0
  wires:
  y0/1 -> Mux/2
  S-function/1 -> table out/1
  x0/1 -> Mux/1
  Mux/1 -> S-function/1

== system BD_PAR_AUTO_base_model/fuel converter  <fc>/fuel use and EO emis Configurable Subsystem/fuel use and EO emis/fc temp correct/fc temp correct Variable Correction Factors (Map Based)/PM factor cold-to-hot ==
  x0 : Inport
  y0 : Inport  Port=2
  Mux : Mux  Inputs=2
  S-function : S-Function  FunctionName=sftable2  Parameters=xindex, yindex, table  SFunctionDeploymentMode=off  EnableBusSupport=off
  table out : Outport  InitialOutput=0
  wires:
  y0/1 -> Mux/2
  S-function/1 -> table out/1
  x0/1 -> Mux/1
  Mux/1 -> S-function/1

== system BD_PAR_AUTO_base_model/fuel converter  <fc>/fuel use and EO emis Configurable Subsystem/fuel use and EO emis/fc temp correct/fc temp correct Variable Correction Factors (Map Based)/fuel factor cold-to-hot ==
  x0 : Inport
  y0 : Inport  Port=2
  Mux : Mux  Inputs=2
  S-function : S-Function  FunctionName=sftable2  Parameters=xindex, yindex, table  SFunctionDeploymentMode=off  EnableBusSupport=off
  table out : Outport  InitialOutput=0
  wires:
  y0/1 -> Mux/2
  S-function/1 -> table out/1
  x0/1 -> Mux/1
  Mux/1 -> S-function/1

== system BD_PAR_AUTO_base_model/mechanical accessory loads <acc>/Mechanical Accessory Loads v2 <acc>/backward model/mechanical accessories (Nm)/Mechanical Accessories: Const Mech Var Elect/Elec Aux Loads 14V Pwr ==
  BrakeLights : Subsystem
  Constant : Constant  Value=0
  Constant1 : Constant  Value=vinf.AuxLoadsOn
  Engine : Subsystem
  ExternalLights : Subsystem
  FrontHVAC : Subsystem
  FrontWipers : Subsystem
  HeatedSeats : Subsystem
  Misc : Subsystem
  RadiatorCoolingFan : Subsystem
  Radio : Subsystem
  RearDefrost : Subsystem
  RearHVAC : Subsystem
  RearWipers : Subsystem
  Starter : Subsystem
  Sum : Sum  Inputs=++++++++++++++  InputSameDT=on  SaturateOnIntegerOverflow=on  OutDataTypeStr=Inherit: Same as first input
  Switch : Switch  Threshold=.5
  TurnSignals : Subsystem
  Out1 : Outport
  wires:
  Switch/1 -> Out1/1
  Sum/1 -> Switch/1
  Constant/1 -> Switch/3
  Constant1/1 -> Switch/2
  RearDefrost/1(Out1) -> Sum/1
  HeatedSeats/1(Out1) -> Sum/2
  Radio/1(Out1) -> Sum/3
  RearWipers/1(Out1) -> Sum/4
  FrontWipers/1(Out1) -> Sum/5
  TurnSignals/1(Out1) -> Sum/6
  Misc/1(Out1) -> Sum/7
  FrontHVAC/1(Out1) -> Sum/8
  RearHVAC/1(Out1) -> Sum/9
  Engine/1(Out1) -> Sum/10
  ExternalLights/1(Out1) -> Sum/11
  RadiatorCoolingFan/1(Out1) -> Sum/12
  BrakeLights/1(Out1) -> Sum/13
  Starter/1(Out1) -> Sum/14

== system BD_PAR_AUTO_base_model/mechanical accessory loads <acc>/Mechanical Accessory Loads v2 <acc>/backward model/mechanical accessories (Nm)/Mechanical Accessories: Const Mech Var Elect/Elec Aux Loads HiV Pwr ==
  Constant : Constant  Value=0
  Constant1 : Constant  Value=vinf.AuxLoadsOn
  CurrentLoad1 : Subsystem
  PowerLoad1 : Subsystem
  PowerLoad2 : Subsystem
  PowerLoad3 : Subsystem
  SpeedLoad1 : Subsystem
  Starter : Subsystem
  Sum : Sum  Inputs=++++++  InputSameDT=on  SaturateOnIntegerOverflow=on  OutDataTypeStr=Inherit: Same as first input
  Switch : Switch  Threshold=.5
  Out1 : Outport
  wires:
  Sum/1 -> Switch/1
  Starter/1(Out1) -> Sum/6
  SpeedLoad1/1(Out1) -> Sum/5
  CurrentLoad1/1(Out1) -> Sum/4
  PowerLoad3/1(Out1) -> Sum/3
  PowerLoad2/1(Out1) -> Sum/2
  PowerLoad1/1(Out1) -> Sum/1
  Constant1/1 -> Switch/2
  Constant/1 -> Switch/3
  Switch/1 -> Out1/1

== system BD_PAR_AUTO_base_model/mechanical accessory loads <acc>/Mechanical Accessory Loads v2 <acc>/backward model/mechanical accessories (Nm)/Mechanical Accessories: Const Mech Var Elect/accessory mechanical torque and power calcs (Nm) ==
  note: acc_call is a "function call" to the
      | accessory block. That block makes
      | a return (acc_return) which is captured below.
  w_APU : Inport
  "accessorie loads \"function\" return values" : Inport  Port=2
  (Nm) : Product  Inputs=*/  InputSameDT=on  RndMeth=Zero  SaturateOnIntegerOverflow=on  OutDataTypeStr=Inherit: Same as first input
  (Nm)1 : Product  Inputs=/*  InputSameDT=on  RndMeth=Zero  SaturateOnIntegerOverflow=on  OutDataTypeStr=Inherit: Same as first input
  (W) : Product  Inputs=*/  InputSameDT=on  RndMeth=Zero  SaturateOnIntegerOverflow=on  OutDataTypeStr=Inherit: Same as first input
  (W)1 : Product  Inputs=*/  InputSameDT=on  RndMeth=Zero  SaturateOnIntegerOverflow=on  OutDataTypeStr=Inherit: Same as first input
  Constant1 : Constant  Value=acc_mech_eff
  Constant2 : Constant  Value=load_on
  Constant5 : Constant  Value=acc_elec_eff
  Demux : Demux  Outputs=3
      settings: DisplayOption=none
  Product : Product  InputSameDT=on  RndMeth=Zero  SaturateOnIntegerOverflow=on  OutDataTypeStr=Inherit: Same as first input
  Product3 : Product  InputSameDT=on  RndMeth=Zero  SaturateOnIntegerOverflow=on  OutDataTypeStr=Inherit: Same as first input
  Sum : Sum  InputSameDT=on  SaturateOnIntegerOverflow=on  OutDataTypeStr=Inherit: Same as first input
  Sum1 : Sum  InputSameDT=on  SaturateOnIntegerOverflow=on  OutDataTypeStr=Inherit: Same as first input
  T_acc : Outport  InitialOutput=0
  P_acc : Outport  Port=2  InitialOutput=0
  wires:
  [acc_elec_pwr] -> (W)1/1
  w_APU/1 -> (Nm)/2, Product/2, (Nm)1/1
  [acc_mech_trq] -> Sum/1
  Constant2/1 -> Product3/1
  Product3/1 -> Sum1/2
  (Nm)1/1 -> Product3/2
  (W)1/1 -> (Nm)1/2
  Constant5/1 -> (W)1/2
  Sum1/1 -> T_acc/1, Product/1
  Sum/1 -> Sum1/1
  (Nm)/1 -> Sum/2
  [acc_mech_pwr] -> (W)/1
  Constant1/1 -> (W)/2
  (W)/1 -> (Nm)/1
  Product/1 -> P_acc/1
  Demux/2 -> [acc_mech_trq]
  Demux/1 -> [acc_mech_pwr]
  Demux/3 -> [acc_elec_pwr]
  "accessorie loads \"function\" return values"/1 -> Demux/1

== system BD_PAR_AUTO_base_model/<vc> par auto/gearbox control for use w/ AT/Speed Dependent Shifting/shifting/time since last shift/timer/no-lag Reset Integrator ==
  in_1 : Inport
  in_2 : Inport  Port=2
  in_3 : Inport  Port=3
  Constant : Constant  Value=0
  Memory : Memory  InitialCondition=initval
  Product : Product  InputSameDT=on  RndMeth=Zero  SaturateOnIntegerOverflow=on  OutDataTypeStr=Inherit: Same as first input
  Sum : Sum  InputSameDT=on  SaturateOnIntegerOverflow=on  OutDataTypeStr=Inherit: Same as first input
  Switch : Switch  Threshold=eps
  dt : Subsystem
  in_2==0 : RelationalOperator  Operator===  RndMeth=Nearest  InputSameDT=on
  out_1 : Outport  InitialOutput=0
  wires:
  Constant/1 -> in_2==0/2
  in_2==0/1 -> Switch/2
  Switch/1 -> Memory/1, out_1/1
  Sum/1 -> Switch/1
  Memory/1 -> Sum/1
  Product/1 -> Sum/2
  dt/1(out_1) -> Product/1
  in_1/1 -> Product/2
  in_2/1 -> in_2==0/1
  in_3/1 -> Switch/3

== system BD_PAR_AUTO_base_model/<vc> par auto/gearbox control for use w/ AT/Speed Dependent Shifting/shifting1/time since last shift/timer/no-lag Reset Integrator ==
  in_1 : Inport
  in_2 : Inport  Port=2
  in_3 : Inport  Port=3
  Constant : Constant  Value=0
  Memory : Memory  InitialCondition=initval
  Product : Product  InputSameDT=on  RndMeth=Zero  SaturateOnIntegerOverflow=on  OutDataTypeStr=Inherit: Same as first input
  Sum : Sum  InputSameDT=on  SaturateOnIntegerOverflow=on  OutDataTypeStr=Inherit: Same as first input
  Switch : Switch  Threshold=eps
  dt : Subsystem
  in_2==0 : RelationalOperator  Operator===  RndMeth=Nearest  InputSameDT=on
  out_1 : Outport  InitialOutput=0
  wires:
  Constant/1 -> in_2==0/2
  in_2==0/1 -> Switch/2
  Switch/1 -> Memory/1, out_1/1
  Sum/1 -> Switch/1
  Memory/1 -> Sum/1
  Product/1 -> Sum/2
  dt/1(out_1) -> Product/1
  in_1/1 -> Product/2
  in_2/1 -> in_2==0/1
  in_3/1 -> Switch/3

== system BD_PAR_AUTO_base_model/<vc> par auto/gearbox control for use w/ AT/shifting1/time since last shift/timer/no-lag Reset Integrator/dt ==
  Clock : Clock
  Memory1 : Memory  InitialCondition=-1
  Sum1 : Sum  Inputs=+-  InputSameDT=on  SaturateOnIntegerOverflow=on  OutDataTypeStr=Inherit: Same as first input
  out_1 : Outport  InitialOutput=0
  wires:
  Sum1/1 -> out_1/1
  Memory1/1 -> Sum1/2
  Clock/1 -> Memory1/1, Sum1/1

== system BD_PAR_AUTO_base_model/electric acc loads <acc>/Electrical Accessory Loads v2 <acc>/backward model/electrical accessories (W)/Electrical Accessories: Time Variable/Elec Aux Loads 14V Pwr/BrakeLights ==
  Average Watts : Constant  Value=vinf.AuxLoads.BrakeLights.AverageWatts
  Constant : Constant  Value=0
  Constant1 : Constant
  On : Constant  Value=vinf.AuxLoads.BrakeLights.On
  Product : Product  Inputs=4  InputSameDT=on  RndMeth=Zero  SaturateOnIntegerOverflow=on  OutDataTypeStr=Inherit: Same as first input
  Switch : Switch
  Out1 : Outport
  wires:
  Switch/1 -> Product/2
  On/1 -> Product/1
  [key_on] -> Product/3
  Average Watts/1 -> Product/4
  Constant1/1 -> Switch/3
  [F_req] -> Switch/2
  Constant/1 -> Switch/1
  Product/1 -> Out1/1
